simulink model "stage4_packetize"  (R2012b)
settings: Solver=FixedStepDiscrete  SolverMode=SingleTasking  StartTime=0.0  StopTime=T  RelTol=1e-3
libraries: xbsIndex_r4 x23, unit_testing x7, r2daq_blocks x1, xps_library x1
settings Model: Creator=ayoung  LastModifiedBy=ayoung
settings DebuggingCC: InheritedTsInSrcMsg=none

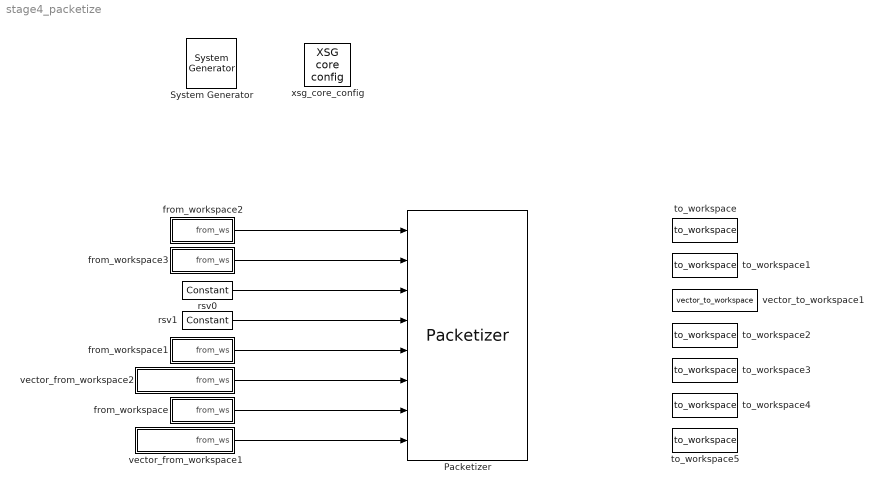
== system stage4_packetize ==
  " System Generator" : xbsIndex_r4/ System Generator  Tag=genX  xilinxfamily=Kintex7  part=xc7k325t  speed=-3  package=fbg676  synthesis_tool=XST  clock_wrapper=Clock Enables  directory=./netlist  proj_type=Project Navigator  Synth_file=XST Defaults  Impl_file=ISE Defaults  testbench=off  simulink_period=1  sysclk_period=10  dcm_input_clock_period=10  incr_netlist=off  trim_vbits=Everywhere in SubSystem  dbl_ovrd=According to Block Masks  core_generation=According to Block Masks  run_coregen=off  deprecated_control=off  eval_field=0  block_type=sysgen
  Packetizer : r2daq_blocks/Packetizer  N_fft=8192  frames_per_batch=390625  IF_ID=1  Digital_ID=3
      link override ud0/io_delay: latency=0  reg_retiming=on
      link override ud1/io_delay: latency=0  reg_retiming=on
  from_workspace : Subsystem  AncestorBlock=unit_testing/from_workspace  mask(from_workspace){n_bits=1, bin_pt=0, arith_type=2, var_name=fsync_in}
      mask prompts: n_bits "Number of bits"; bin_pt "Binary point"; arith_type "Arithmetic type (ufix=0, fix=1, bool=2)"; var_name "Variable name"
      mask init:
      | blk = from_workspace_init(gcb,...
      |     'n_bits', n_bits,...
      |     'bin_pt',bin_pt,...
      |     'arith_type',arith_type,...
      |     'var_name',var_name);
      mask Display:
      | color('white');
      | text(0.5,0.5,get_param(gcb,'var_name'),'HorizontalAlignment','center');
  from_workspace1 : Subsystem  AncestorBlock=unit_testing/from_workspace  mask(from_workspace){n_bits=1, bin_pt=0, arith_type=2, var_name=tsync_in}
      mask prompts: n_bits "Number of bits"; bin_pt "Binary point"; arith_type "Arithmetic type (ufix=0, fix=1, bool=2)"; var_name "Variable name"
      mask init:
      | blk = from_workspace_init(gcb,...
      |     'n_bits', n_bits,...
      |     'bin_pt',bin_pt,...
      |     'arith_type',arith_type,...
      |     'var_name',var_name);
      mask Display:
      | color('white');
      | text(0.5,0.5,get_param(gcb,'var_name'),'HorizontalAlignment','center');
  from_workspace2 : Subsystem  AncestorBlock=unit_testing/from_workspace  mask(from_workspace){n_bits=1, bin_pt=0, arith_type=2, var_name=rst}
      mask prompts: n_bits "Number of bits"; bin_pt "Binary point"; arith_type "Arithmetic type (ufix=0, fix=1, bool=2)"; var_name "Variable name"
      mask init:
      | blk = from_workspace_init(gcb,...
      |     'n_bits', n_bits,...
      |     'bin_pt',bin_pt,...
      |     'arith_type',arith_type,...
      |     'var_name',var_name);
      mask Display:
      | color('white');
      | text(0.5,0.5,get_param(gcb,'var_name'),'HorizontalAlignment','center');
  from_workspace3 : Subsystem  AncestorBlock=unit_testing/from_workspace  mask(from_workspace){n_bits=32, bin_pt=0, arith_type=0, var_name=ut}
      mask prompts: n_bits "Number of bits"; bin_pt "Binary point"; arith_type "Arithmetic type (ufix=0, fix=1, bool=2)"; var_name "Variable name"
      mask init:
      | blk = from_workspace_init(gcb,...
      |     'n_bits', n_bits,...
      |     'bin_pt',bin_pt,...
      |     'arith_type',arith_type,...
      |     'var_name',var_name);
      mask Display:
      | color('white');
      | text(0.5,0.5,get_param(gcb,'var_name'),'HorizontalAlignment','center');
  rsv0 : xbsIndex_r4/Constant  const=0  gui_display_data_type=Fixed-point  arith_type=Unsigned  n_bits=64  bin_pt=0  preci_type=Single  exp_width=8  frac_width=24  explicit_period=on  period=1  equ=P=C  opselect=C  inp2=PCIN>>17  opr=+  inp1=P  carry=CIN  dbl_ovrd=off  block_type=constant
  rsv1 : xbsIndex_r4/Constant  const=0  gui_display_data_type=Fixed-point  arith_type=Unsigned  n_bits=64  bin_pt=0  preci_type=Single  exp_width=8  frac_width=24  explicit_period=on  period=1  equ=P=C  opselect=C  inp2=PCIN>>17  opr=+  inp1=P  carry=CIN  dbl_ovrd=off  block_type=constant
  to_workspace : unit_testing/to_workspace  var_name=tx_eof
  to_workspace1 : unit_testing/to_workspace  var_name=tx_valid
  to_workspace2 : unit_testing/to_workspace  var_name=ffifo_full
  to_workspace3 : unit_testing/to_workspace  var_name=ffifo_empty
  to_workspace4 : unit_testing/to_workspace  var_name=tfifo_full
  to_workspace5 : unit_testing/to_workspace  var_name=tfifo_empty
  vector_from_workspace1 : Subsystem  AncestorBlock=unit_testing/vector_from_workspace  mask(vector_from_workspace){n_in=2, n_bits=8, bin_pt=7, arith_type=1, var_pfx=fdin_c}
      mask prompts: n_in "Number of inputs"; n_bits "Input width"; bin_pt "Binary point position"; arith_type "Arithmetic type (ufix=0, fix=1, bool=2)"; var_pfx "Variable name prefix"
      mask init:
      | blk = vector_from_workspace_init(gcb,...
      |     'n_in',n_in,...
      |     'n_bits',n_bits,...
      |     'bin_pt',bin_pt,...
      |     'arith_type',arith_type,...
      |     'var_pfx',var_pfx);
      mask Display:
      | color('white');
      | var_pfx = get_param(gcb,'var_pfx');
      | n_1 = 1;
      | n_N = str2num(get_param(gcb,'n_in'));
      | text(0.5,0.5,sprintf('%s_[%d..%d]',var_pfx,n_1,n_N),'HorizontalAlignment','center');
  vector_from_workspace2 : Subsystem  AncestorBlock=unit_testing/vector_from_workspace  mask(vector_from_workspace){n_in=2, n_bits=8, bin_pt=7, arith_type=1, var_pfx=tdin_c}
      mask prompts: n_in "Number of inputs"; n_bits "Input width"; bin_pt "Binary point position"; arith_type "Arithmetic type (ufix=0, fix=1, bool=2)"; var_pfx "Variable name prefix"
      mask init:
      | blk = vector_from_workspace_init(gcb,...
      |     'n_in',n_in,...
      |     'n_bits',n_bits,...
      |     'bin_pt',bin_pt,...
      |     'arith_type',arith_type,...
      |     'var_pfx',var_pfx);
      mask Display:
      | color('white');
      | var_pfx = get_param(gcb,'var_pfx');
      | n_1 = 1;
      | n_N = str2num(get_param(gcb,'n_in'));
      | text(0.5,0.5,sprintf('%s_[%d..%d]',var_pfx,n_1,n_N),'HorizontalAlignment','center');
  vector_to_workspace1 : unit_testing/vector_to_workspace  n_out=8  n_bits=8  bin_pt=7  arith_type=1  var_pfx=dout_x4_c
  xsg_core_config : xps_library/XSG core config  Tag=xps:xsg  hw_sys=ROACH2:sx475t  clk_src=adc0_clk  ROACH_clk_src=sys_clk  ROACH2_clk_src=adc0_clk  MKDIG_clk_src=sys_clk  clk_rate=200  sample_period=1  synthesis_tool=XST
  wires:
  vector_from_workspace2/1(from_ws) -> Packetizer/6
  rsv0/1 -> Packetizer/3
  rsv1/1 -> Packetizer/4
  vector_from_workspace1/1(from_ws) -> Packetizer/8
  from_workspace2/1(from_ws) -> Packetizer/1
  from_workspace3/1(from_ws) -> Packetizer/2
  from_workspace1/1(from_ws) -> Packetizer/5
  from_workspace/1(from_ws) -> Packetizer/7

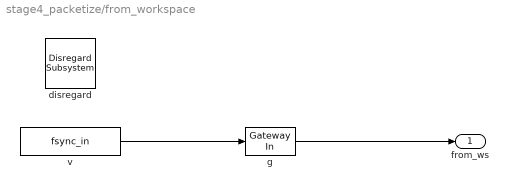
== system stage4_packetize/from_workspace ==
  disregard : xbsIndex_r4/Disregard Subsystem  Tag=discardX  block_type=disregard
  g : xbsIndex_r4/Gateway In  gui_display_data_type=Fixed-point  arith_type=Boolean  n_bits=1  bin_pt=0  preci_type=Single  exp_width=8  frac_width=24  quantization="Round  (unbiased: +/- Inf)"  overflow=Saturate  period=1  dbl_ovrd=off  timing_constraint=None  locs_specified=off  LOCs={}  UseAsADC=off  ADCChannel='1'  inherit_from_input=off  hdl_port=on  block_type=gatewayin
  v : FromWorkspace  VariableName=fsync_in  SampleTime=0
  from_ws : Outport
  wires:
  v/1 -> g/1
  g/1 -> from_ws/1

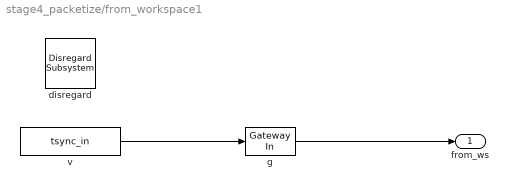
== system stage4_packetize/from_workspace1 ==
  disregard : xbsIndex_r4/Disregard Subsystem  Tag=discardX  block_type=disregard
  g : xbsIndex_r4/Gateway In  gui_display_data_type=Fixed-point  arith_type=Boolean  n_bits=1  bin_pt=0  preci_type=Single  exp_width=8  frac_width=24  quantization="Round  (unbiased: +/- Inf)"  overflow=Saturate  period=1  dbl_ovrd=off  timing_constraint=None  locs_specified=off  LOCs={}  UseAsADC=off  ADCChannel='1'  inherit_from_input=off  hdl_port=on  block_type=gatewayin
  v : FromWorkspace  VariableName=tsync_in  SampleTime=0
  from_ws : Outport
  wires:
  v/1 -> g/1
  g/1 -> from_ws/1

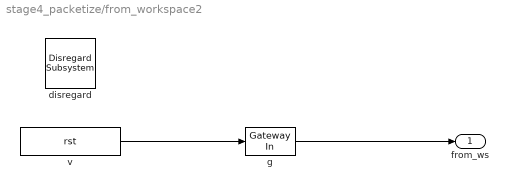
== system stage4_packetize/from_workspace2 ==
  disregard : xbsIndex_r4/Disregard Subsystem  Tag=discardX  block_type=disregard
  g : xbsIndex_r4/Gateway In  gui_display_data_type=Fixed-point  arith_type=Boolean  n_bits=1  bin_pt=0  preci_type=Single  exp_width=8  frac_width=24  quantization="Round  (unbiased: +/- Inf)"  overflow=Saturate  period=1  dbl_ovrd=off  timing_constraint=None  locs_specified=off  LOCs={}  UseAsADC=off  ADCChannel='1'  inherit_from_input=off  hdl_port=on  block_type=gatewayin
  v : FromWorkspace  VariableName=rst  SampleTime=0
  from_ws : Outport
  wires:
  v/1 -> g/1
  g/1 -> from_ws/1

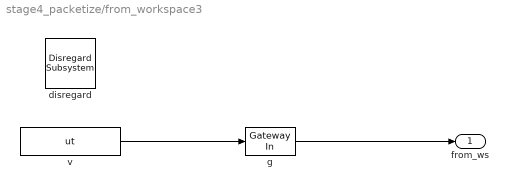
== system stage4_packetize/from_workspace3 ==
  disregard : xbsIndex_r4/Disregard Subsystem  Tag=discardX  block_type=disregard
  g : xbsIndex_r4/Gateway In  gui_display_data_type=Fixed-point  arith_type=Unsigned  n_bits=32  bin_pt=0  preci_type=Single  exp_width=8  frac_width=24  quantization="Round  (unbiased: +/- Inf)"  overflow=Saturate  period=1  dbl_ovrd=off  timing_constraint=None  locs_specified=off  LOCs={}  UseAsADC=off  ADCChannel='1'  inherit_from_input=off  hdl_port=on  block_type=gatewayin
  v : FromWorkspace  VariableName=ut  SampleTime=0
  from_ws : Outport
  wires:
  v/1 -> g/1
  g/1 -> from_ws/1

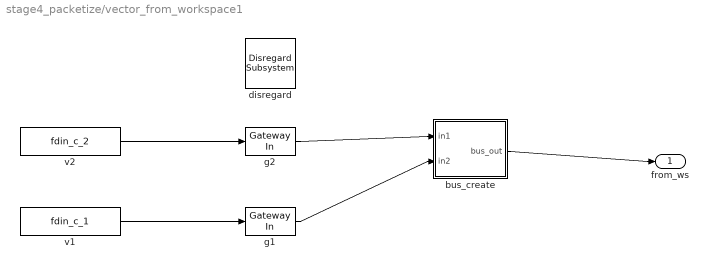
== system stage4_packetize/vector_from_workspace1 ==
  bus_create : Subsystem  AncestorBlock=casper_library_flow_control/bus_create  mask(bus_create){inputNum=2}
      mask prompts: inputNum "Number of inputs:"
      mask init:
      | bus_create_init(gcb,...
      |     'inputNum', inputNum);
  disregard : xbsIndex_r4/Disregard Subsystem  Tag=discardX  block_type=disregard
  g1 : xbsIndex_r4/Gateway In  gui_display_data_type=Fixed-point  arith_type="Signed  (2's comp)"  n_bits=8  bin_pt=7  preci_type=Single  exp_width=8  frac_width=24  quantization="Round  (unbiased: +/- Inf)"  overflow=Saturate  period=1  dbl_ovrd=off  timing_constraint=None  locs_specified=off  LOCs={}  UseAsADC=off  ADCChannel='1'  inherit_from_input=off  hdl_port=on  block_type=gatewayin
  g2 : xbsIndex_r4/Gateway In  gui_display_data_type=Fixed-point  arith_type="Signed  (2's comp)"  n_bits=8  bin_pt=7  preci_type=Single  exp_width=8  frac_width=24  quantization="Round  (unbiased: +/- Inf)"  overflow=Saturate  period=1  dbl_ovrd=off  timing_constraint=None  locs_specified=off  LOCs={}  UseAsADC=off  ADCChannel='1'  inherit_from_input=off  hdl_port=on  block_type=gatewayin
  v1 : FromWorkspace  VariableName=fdin_c_1
  v2 : FromWorkspace  VariableName=fdin_c_2
  from_ws : Outport
  wires:
  v2/1 -> g2/1
  v1/1 -> g1/1
  g2/1 -> bus_create/1(in1)
  g1/1 -> bus_create/2(in2)
  bus_create/1(bus_out) -> from_ws/1

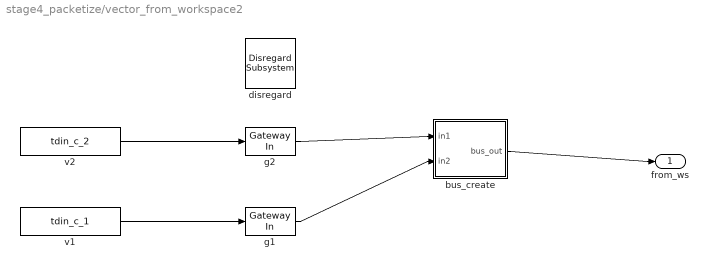
== system stage4_packetize/vector_from_workspace2 ==
  bus_create : Subsystem  AncestorBlock=casper_library_flow_control/bus_create  mask(bus_create){inputNum=2}
      mask prompts: inputNum "Number of inputs:"
      mask init:
      | bus_create_init(gcb,...
      |     'inputNum', inputNum);
  disregard : xbsIndex_r4/Disregard Subsystem  Tag=discardX  block_type=disregard
  g1 : xbsIndex_r4/Gateway In  gui_display_data_type=Fixed-point  arith_type="Signed  (2's comp)"  n_bits=8  bin_pt=7  preci_type=Single  exp_width=8  frac_width=24  quantization="Round  (unbiased: +/- Inf)"  overflow=Saturate  period=1  dbl_ovrd=off  timing_constraint=None  locs_specified=off  LOCs={}  UseAsADC=off  ADCChannel='1'  inherit_from_input=off  hdl_port=on  block_type=gatewayin
  g2 : xbsIndex_r4/Gateway In  gui_display_data_type=Fixed-point  arith_type="Signed  (2's comp)"  n_bits=8  bin_pt=7  preci_type=Single  exp_width=8  frac_width=24  quantization="Round  (unbiased: +/- Inf)"  overflow=Saturate  period=1  dbl_ovrd=off  timing_constraint=None  locs_specified=off  LOCs={}  UseAsADC=off  ADCChannel='1'  inherit_from_input=off  hdl_port=on  block_type=gatewayin
  v1 : FromWorkspace  VariableName=tdin_c_1
  v2 : FromWorkspace  VariableName=tdin_c_2
  from_ws : Outport
  wires:
  v2/1 -> g2/1
  v1/1 -> g1/1
  g2/1 -> bus_create/1(in1)
  g1/1 -> bus_create/2(in2)
  bus_create/1(bus_out) -> from_ws/1

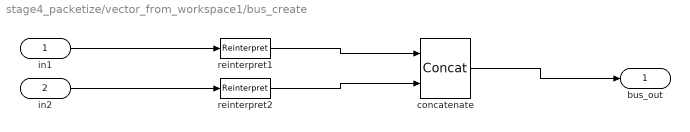
== system stage4_packetize/vector_from_workspace1/bus_create ==
  in1 : Inport
  in2 : Inport  Port=2
  concatenate : xbsIndex_r4/Concat  num_inputs=2  dbl_ovrd=off  block_type=concat
  reinterpret1 : xbsIndex_r4/Reinterpret  force_arith_type=on  arith_type=Unsigned  force_bin_pt=on  bin_pt=0  block_type=reinterpret
      settings: infoedit="Changes signal type without altering the binary representation.   You can changed the signal between signed and unsigned, and relocate the binary point.<br><br>Hardware notes: In hardware this block costs nothing.<br><br>Example:  Suppose the input is 6 bits wide, signed, with 2 fractional bits, and the output is forced to unsigned with 0 fractional bits.  Then an input of -2.0 (1110.00 in binary 2's complement) becomes an output of 56 (111000 in binary)."
  reinterpret2 : xbsIndex_r4/Reinterpret  force_arith_type=on  arith_type=Unsigned  force_bin_pt=on  bin_pt=0  block_type=reinterpret
      settings: infoedit="Changes signal type without altering the binary representation.   You can changed the signal between signed and unsigned, and relocate the binary point.<br><br>Hardware notes: In hardware this block costs nothing.<br><br>Example:  Suppose the input is 6 bits wide, signed, with 2 fractional bits, and the output is forced to unsigned with 0 fractional bits.  Then an input of -2.0 (1110.00 in binary 2's complement) becomes an output of 56 (111000 in binary)."
  bus_out : Outport
  wires:
  concatenate/1 -> bus_out/1
  in1/1 -> reinterpret1/1
  reinterpret1/1 -> concatenate/1
  in2/1 -> reinterpret2/1
  reinterpret2/1 -> concatenate/2

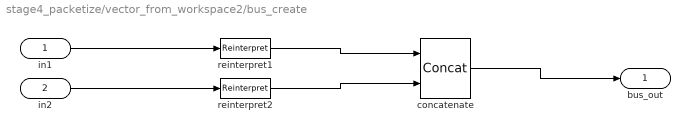
== system stage4_packetize/vector_from_workspace2/bus_create ==
  in1 : Inport
  in2 : Inport  Port=2
  concatenate : xbsIndex_r4/Concat  num_inputs=2  dbl_ovrd=off  block_type=concat
  reinterpret1 : xbsIndex_r4/Reinterpret  force_arith_type=on  arith_type=Unsigned  force_bin_pt=on  bin_pt=0  block_type=reinterpret
      settings: infoedit="Changes signal type without altering the binary representation.   You can changed the signal between signed and unsigned, and relocate the binary point.<br><br>Hardware notes: In hardware this block costs nothing.<br><br>Example:  Suppose the input is 6 bits wide, signed, with 2 fractional bits, and the output is forced to unsigned with 0 fractional bits.  Then an input of -2.0 (1110.00 in binary 2's complement) becomes an output of 56 (111000 in binary)."
  reinterpret2 : xbsIndex_r4/Reinterpret  force_arith_type=on  arith_type=Unsigned  force_bin_pt=on  bin_pt=0  block_type=reinterpret
      settings: infoedit="Changes signal type without altering the binary representation.   You can changed the signal between signed and unsigned, and relocate the binary point.<br><br>Hardware notes: In hardware this block costs nothing.<br><br>Example:  Suppose the input is 6 bits wide, signed, with 2 fractional bits, and the output is forced to unsigned with 0 fractional bits.  Then an input of -2.0 (1110.00 in binary 2's complement) becomes an output of 56 (111000 in binary)."
  bus_out : Outport
  wires:
  concatenate/1 -> bus_out/1
  in1/1 -> reinterpret1/1
  reinterpret1/1 -> concatenate/1
  in2/1 -> reinterpret2/1
  reinterpret2/1 -> concatenate/2
